simulink model "s0319"  (Simulink 6.0)
settings: Solver=ode3  SolverMode=SingleTasking  StartTime=0.0  StopTime=900  FixedStep=1  MaxStep=1  RelTol=1e-3  AbsTol=1e-6
values from neighbouring files (symbols this model uses):
  nen = Gs.den{1}    [m0251.m]    (also in m0252.m; m0256.m; m0258.m; m0304.m = G.den{1})
  PT2nen1 = G.den{1}    [m0319.m]
  PT2nen2 = G.den{1}    [m0319.m]
  PT2zae1 = G.num{1}    [m0319.m]
  PT2zae2 = G.num{1}    [m0319.m]
  ydach = 1    [m0305.m]    (also in m0306.m; m0311.m; m0312b.m; m0313.m)
  zae = Gs.num{1}    [m0251.m]    (also in m0252.m; m0256.m; m0258.m; m0304.m = G.num{1})
settings Model: LastModifiedBy=Froriep
settings DataIOCC: LimitDataPoints=off  SaveOutput=off  SaveTime=off
settings OptimizationCC: BooleanDataType=off
settings DebuggingCC: SolverPrmCheckMsg=none
settings HardwareCC: TargetUnknown=on
settings GRTTargetCC: ModelReferenceCompliant=off  MatFileLogging=off

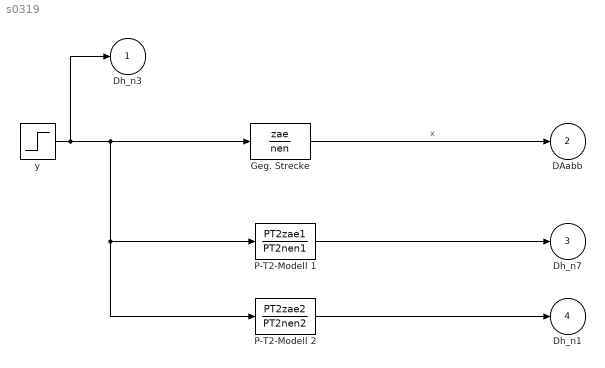
== system s0319 ==
  Geg. Strecke : TransferFcn  Numerator=zae  Denominator=nen
  P-T2-Modell 1 : TransferFcn  Numerator=PT2zae1  Denominator=PT2nen1
  P-T2-Modell 2 : TransferFcn  Numerator=PT2zae2  Denominator=PT2nen2
  y : Step  Time=0  After=ydach  SampleTime=0
  Dh_n3 : Outport
  DAabb : Outport  Port=2
  Dh_n7 : Outport  Port=3
  Dh_n1 : Outport  Port=4
  wires:
  y/1 -> Dh_n3/1, Geg. Strecke/1, P-T2-Modell 1/1, P-T2-Modell 2/1
  P-T2-Modell 1/1 -> Dh_n7/1
  Geg. Strecke/1 -> DAabb/1  "x"
  P-T2-Modell 2/1 -> Dh_n1/1
